simulink model "Simu_Autopilot_2015_updated"  (R2015a)
settings: Solver=ode15s  StartTime=0.0  StopTime=240  RelTol=1e-3
InitFcn:
  | clear all
  | addpath('../parameters/')
  | aerosonde_parameters
  | simulation_parameters
  | wind_parameters
  | compute_autopilot_gains
undefined symbols (not defined in the file or in its folder): autopilot, drawAircraft, forces_moments, plotmavstatevariables, SIM, UAV, WIND
libraries: simulink x6
settings Model: CovHtmlReporting=off  CovSFcnEnable=off  Creator=beard  LastModifiedBy=h1huang
settings DataIOCC: SignalLoggingSaveFormat=ModelDataLogs
settings OptimizationCC: ExpressionDepthLimit=2147483647  InitFltsAndDblsToZero=on
settings DebuggingCC: UnderspecifiedInitializationDetection=Classic  MergeDetectMultiDrivingBlocksExec=none  SolverPrmCheckMsg=warning  FcnCallInpInsideContextMsg=EnableAllAsWarning  StateNameClashWarn=warning
settings GRTTargetCC: CombineOutputUpdateFcns=off  GRTInterface=on

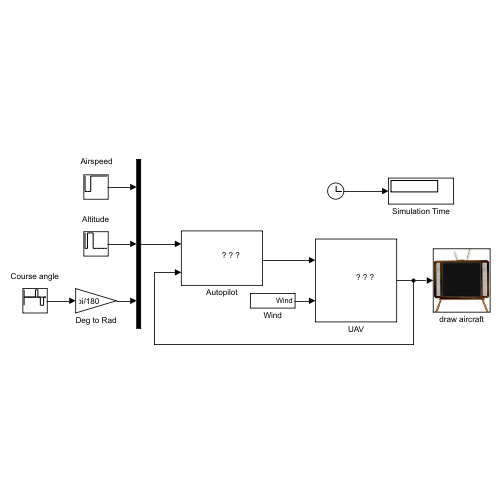
[thumbnail: Simulink's stored preview of the top-level diagram]
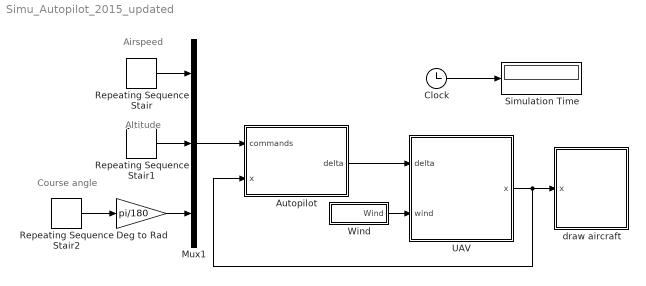
== system Simu_Autopilot_2015_updated ==
  note: Altitude
  note: Airspeed
  note: Course angle
  Autopilot : Subsystem
      mask Display: image(imread('kestrel.jpg'))
  Clock : Clock
  Deg to Rad : Gain  Gain=pi/180
  Mux1 : Mux  Inputs=3
  Repeating Sequence Stair : simulink/Sources/Repeating Sequence Stair  OutValues=[25 25 30 30 30 30 30 30].'  tsamp=25  OutMin=[]  OutMax=[]  OutDataTypeStr=double  OutputDataTypeScalingMode=double  OutDataType=fixdt(0,8)  ConRadixGroup=Best Precision: Vector-wise  OutScaling=2^-12
  Repeating Sequence Stair1 : simulink/Sources/Repeating Sequence Stair  OutValues=[30 40 40 30 30 30 30 30].'  tsamp=25  OutMin=[]  OutMax=[]  OutDataTypeStr=double  OutputDataTypeScalingMode=double  OutDataType=fixdt(0,8)  ConRadixGroup=Best Precision: Vector-wise  OutScaling=2^-12
  Repeating Sequence Stair2 : simulink/Sources/Repeating Sequence Stair  OutValues=[0 0 0 0 10 0 -10 0].'  tsamp=25  OutMin=[]  OutMax=[]  OutDataTypeStr=double  OutputDataTypeScalingMode=double  OutDataType=fixdt(0,8)  ConRadixGroup=Best Precision: Vector-wise  OutScaling=2^-12
  Simulation Time : Display
  UAV : Subsystem
      mask Display: image(imread('batcam.png'))
  Wind : Subsystem
  draw aircraft : Subsystem
      mask Display: image(imread('tv.jpg'))
  wires:
  Clock/1 -> Simulation Time/1
  Wind/1(Wind) -> UAV/2(wind)
  UAV/1(x) -> Autopilot/2(x), draw aircraft/1(x)
  Autopilot/1(delta) -> UAV/1(delta)
  Mux1/1 -> Autopilot/1(commands)
  Deg to Rad/1 -> Mux1/3
  Repeating Sequence Stair1/1 -> Mux1/2
  Repeating Sequence Stair2/1 -> Deg to Rad/1
  Repeating Sequence Stair/1 -> Mux1/1

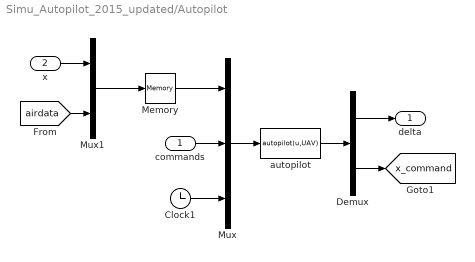
== system Simu_Autopilot_2015_updated/Autopilot ==
  commands : Inport
  x : Inport  Port=2
  Clock1 : Clock
  Demux : Demux  Outputs=[4;12]
  Memory : Memory
  Mux : Mux  Inputs=3
  Mux1 : Mux  Inputs=2
  autopilot : MATLABFcn  MATLABFcn=autopilot(u,UAV)  OutputDimensions=4+12  SampleTime=SIM.ts_simulation
  delta : Outport
  tag scope: x_command=global
  wires:
  Mux/1 -> autopilot/1
  autopilot/1 -> Demux/1
  Demux/1 -> delta/1
  Demux/2 -> [x_command]
  commands/1 -> Mux/2
  x/1 -> Mux1/1
  [airdata] -> Mux1/2
  Clock1/1 -> Mux/3
  Mux1/1 -> Memory/1
  Memory/1 -> Mux/1

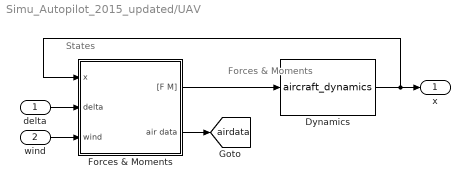
== system Simu_Autopilot_2015_updated/UAV ==
  note: Forces & Moments
  note: States
  delta : Inport
  wind : Inport  Port=2
  Dynamics : S-Function  FunctionName=aircraft_dynamics  Parameters=UAV  SFunctionDeploymentMode=off  EnableBusSupport=off
  Forces & Moments : Subsystem
  x : Outport
  tag scope: airdata=global
  wires:
  Dynamics/1 -> Forces & Moments/1(x), x/1
  Forces & Moments/1("[F M]") -> Dynamics/1
  Forces & Moments/2(air data) -> [airdata]
  delta/1 -> Forces & Moments/2(delta)
  wind/1 -> Forces & Moments/3(wind)

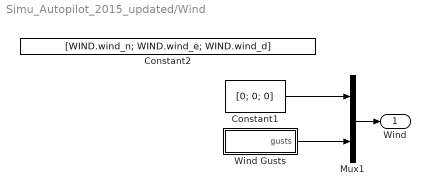
== system Simu_Autopilot_2015_updated/Wind ==
  Constant1 : Constant  Value=[0; 0; 0]
  Constant2 : Constant  Value=[WIND.wind_n; WIND.wind_e; WIND.wind_d]
  Mux1 : Mux  Inputs=2
  Wind Gusts : Subsystem
  Wind : Outport
  wires:
  Mux1/1 -> Wind/1
  Wind Gusts/1(gusts) -> Mux1/2
  Constant1/1 -> Mux1/1

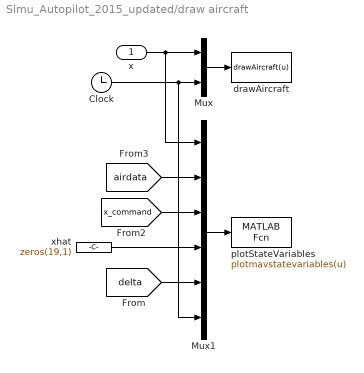
== system Simu_Autopilot_2015_updated/draw aircraft ==
  x : Inport
  Clock : Clock
  Mux : Mux  Inputs=2
  Mux1 : Mux  Inputs=6
  drawAircraft : MATLABFcn  MATLABFcn=drawAircraft(u)  OutputDimensions=0  SampleTime=SIM.ts_plotting
  plotStateVariables : MATLABFcn  MATLABFcn=plotmavstatevariables(u)  OutputDimensions=0  SampleTime=SIM.ts_plotting
  xhat : Constant  Value=zeros(19,1)
  wires:
  Mux/1 -> drawAircraft/1
  x/1 -> Mux1/1, Mux/1
  Clock/1 -> Mux1/6, Mux/2
  Mux1/1 -> plotStateVariables/1
  [x_command] -> Mux1/3
  [delta] -> Mux1/5
  [airdata] -> Mux1/2
  xhat/1 -> Mux1/4

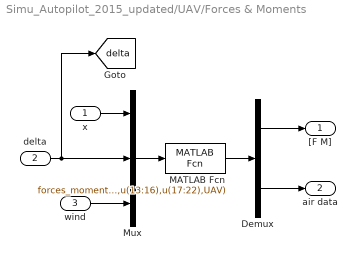
== system Simu_Autopilot_2015_updated/UAV/Forces & Moments ==
  x : Inport
  delta : Inport  Port=2
  wind : Inport  Port=3
  Demux : Demux  Outputs=[6;6]
  MATLAB Fcn : MATLABFcn  MATLABFcn=forces_moments(u(1:12),u(13:16),u(17:22),UAV)  OutputDimensions=12
  Mux : Mux  Inputs=3
  "[F M]" : Outport
  air data : Outport  Port=2
  tag scope: delta=global
  wires:
  Demux/2 -> air data/1
  Mux/1 -> MATLAB Fcn/1
  Demux/1 -> "[F M]"/1
  MATLAB Fcn/1 -> Demux/1
  wind/1 -> Mux/3
  delta/1 -> [delta], Mux/2
  x/1 -> Mux/1

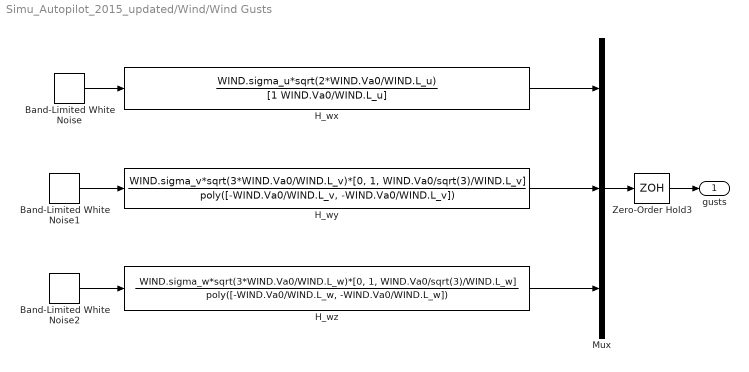
== system Simu_Autopilot_2015_updated/Wind/Wind Gusts ==
  Band-Limited White Noise : simulink/Sources/Band-Limited White Noise  Cov=[0.1]  Ts=SIM.ts_simulation  seed=[23341]
  Band-Limited White Noise1 : simulink/Sources/Band-Limited White Noise  Cov=[0.1]  Ts=SIM.ts_simulation  seed=[23341]
  Band-Limited White Noise2 : simulink/Sources/Band-Limited White Noise  Cov=[0.1]  Ts=SIM.ts_simulation  seed=[23341]
  H_wx : TransferFcn  Numerator=WIND.sigma_u*sqrt(2*WIND.Va0/WIND.L_u)  Denominator=[1 WIND.Va0/WIND.L_u]
  H_wy : TransferFcn  Numerator=WIND.sigma_v*sqrt(3*WIND.Va0/WIND.L_v)*[0, 1, WIND.Va0/sqrt(3)/WIND.L_v]  Denominator=poly([-WIND.Va0/WIND.L_v, -WIND.Va0/WIND.L_v])
  H_wz : TransferFcn  Numerator=WIND.sigma_w*sqrt(3*WIND.Va0/WIND.L_w)*[0, 1, WIND.Va0/sqrt(3)/WIND.L_w]  Denominator=poly([-WIND.Va0/WIND.L_w, -WIND.Va0/WIND.L_w])
  Mux : Mux  Inputs=3
  Zero-Order Hold3 : ZeroOrderHold  SampleTime=SIM.ts_simulation
  gusts : Outport
  wires:
  H_wx/1 -> Mux/1
  Band-Limited White Noise/1 -> H_wx/1
  H_wy/1 -> Mux/2
  Band-Limited White Noise1/1 -> H_wy/1
  H_wz/1 -> Mux/3
  Band-Limited White Noise2/1 -> H_wz/1
  Mux/1 -> Zero-Order Hold3/1
  Zero-Order Hold3/1 -> gusts/1
